simulink model "st_re_3_fig2"  (R2017b)
settings: Solver=VariableStepAuto  StartTime=0.0  StopTime=5  MaxStep=1e-4  RelTol=1e-3
libraries: dsparch4 x2
settings Model: Creator=Administrator  LastModifiedBy=Administrator

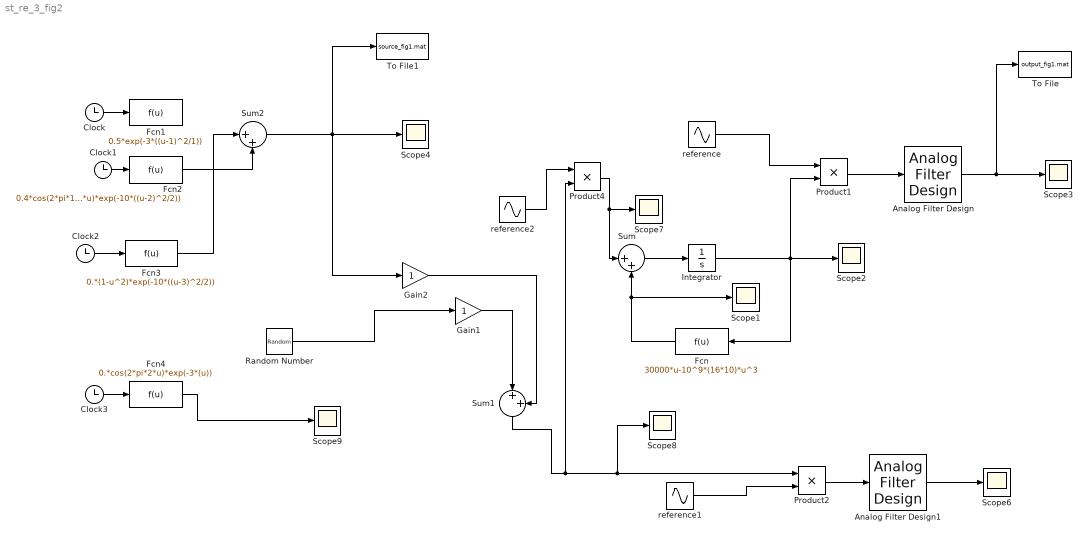
== system st_re_3_fig2 ==
  Analog Filter Design : dsparch4/Analog Filter Design  method=Butterworth  filttype=Lowpass  N=20  Wlo=20  Whi=80  Rp=2  Rs=40
  Analog Filter Design1 : dsparch4/Analog Filter Design  method=Butterworth  filttype=Lowpass  N=8  Wlo=10  Whi=80  Rp=2  Rs=40
  Clock{,1..3} (4 alike) : Clock
  Fcn : Fcn  Expr=30000*u-10^9*(16*10)*u^3
  Fcn1 : Fcn  Expr=0.5*exp(-3*((u-1)^2/1))
  Fcn2 : Fcn  Expr=0.4*cos(2*pi*1*u)*exp(-10*((u-2)^2/2))
  Fcn3 : Fcn  Expr=0.*(1-u^2)*exp(-10*((u-3)^2/2))
  Fcn4 : Fcn  Expr=0.*cos(2*pi*2*u)*exp(-3*(u))
  Gain1 : Gain
  Gain2 : Gain
  Integrator : Integrator
  Product1 : Product
  Product2 : Product
  Product4 : Product
  Random Number : RandomNumber  Variance=4  SampleTime=0.0001
  Scope{1..4,6..9} (8 alike) : Scope
  Sum : Sum  Inputs=|++
  Sum1 : Sum  Inputs=|++
  Sum2 : Sum  Inputs=|++
  To File : ToFile  Filename=output_fig1.mat  MatrixName=output_f1  SaveFormat=Timeseries
  To File1 : ToFile  Filename=source_fig1.mat  MatrixName=source_f1  SaveFormat=Timeseries
  reference : Sin  Amplitude=10  Frequency=1000  Phase=pi/3  SampleTime=0.001
  reference1 : Sin  Amplitude=2  Frequency=1000  Phase=pi/3  SampleTime=0.001
  reference2 : Sin  Amplitude=0.4  Frequency=1000  Phase=pi/3  SampleTime=0.001
  wires:
  Gain1/1 -> Sum1/1
  Fcn/1 -> Sum/2, Scope1/1
  Sum1/1 -> Product4/2, Scope8/1, Product2/1
  Clock/1 -> Fcn1/1
  Clock1/1 -> Fcn2/1
  reference/1 -> Product1/1
  Integrator/1 -> Product1/2, Scope2/1, Fcn/1
  Product1/1 -> Analog Filter Design/1
  Analog Filter Design/1 -> To File/1, Scope3/1
  Sum2/1 -> To File1/1, Gain2/1, Scope4/1
  Clock2/1 -> Fcn3/1
  Product2/1 -> Analog Filter Design1/1
  Analog Filter Design1/1 -> Scope6/1
  reference1/1 -> Product2/2
  Sum/1 -> Integrator/1
  Random Number/1 -> Gain1/1
  reference2/1 -> Product4/1
  Gain2/1 -> Sum1/2
  Product4/1 -> Scope7/1, Sum/1
  Clock3/1 -> Fcn4/1
  Fcn4/1 -> Scope9/1
  Fcn2/1 -> Sum2/2
  Fcn3/1 -> Sum2/1
